simulink model "q1"  (R2022a)
settings: Solver=VariableStepAuto  StartTime=0.0  StopTime=10.0  RelTol=1e-3
undefined symbols (not defined in the file): aphi1, aphi2, g, kdphi, kikai, kpkai, kpphi, Va
settings Model: Creator=Kushal  LastModifiedBy=Kushal

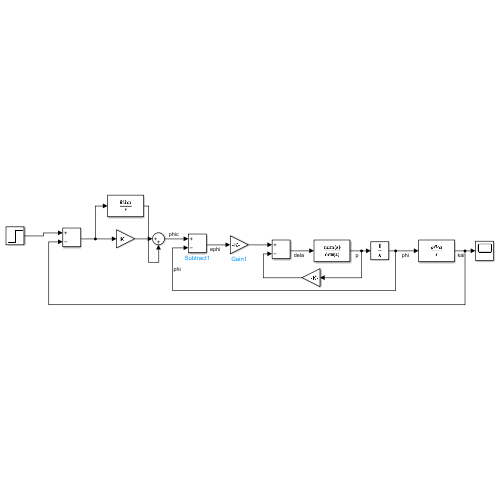
[thumbnail: Simulink's stored preview of the top-level diagram]
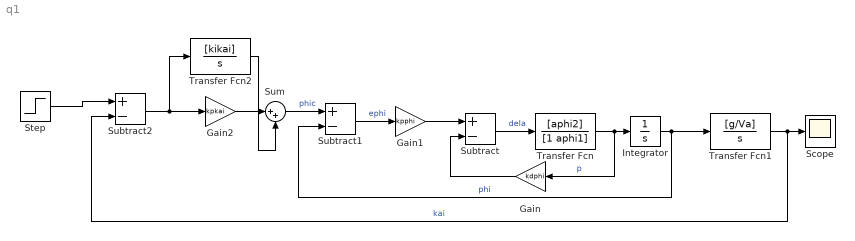
== system q1 ==
  Gain : Gain  Gain=kdphi
  Gain1 : Gain  Gain=kpphi
  Gain2 : Gain  Gain=kpkai
  Integrator : Integrator
  Scope : Scope
  Step : Step  Time=0  SampleTime=0
  Subtract : Sum  Inputs=+-
  Subtract1 : Sum  Inputs=+-
  Subtract2 : Sum  Inputs=+-
  Sum : Sum  Inputs=|++
  Transfer Fcn : TransferFcn  Numerator=[aphi2]  Denominator=[1 aphi1]
  Transfer Fcn1 : TransferFcn  Numerator=[g/Va]  Denominator=[1 0]
  Transfer Fcn2 : TransferFcn  Numerator=[kikai]  Denominator=[1 0]
  wires:
  Transfer Fcn/1 -> Gain/1, Integrator/1  "p"
  Gain/1 -> Subtract/2
  Subtract/1 -> Transfer Fcn/1  "dela"
  Gain1/1 -> Subtract/1
  Subtract1/1 -> Gain1/1  "ephi"
  Integrator/1 -> Transfer Fcn1/1, Subtract1/2  "phi"
  Sum/1 -> Subtract1/1  "phic"
  Transfer Fcn1/1 -> Subtract2/2, Scope/1  "kai"
  Subtract2/1 -> Transfer Fcn2/1, Gain2/1
  Gain2/1 -> Sum/1
  Transfer Fcn2/1 -> Sum/2
  Step/1 -> Subtract2/1
